simulink library "csu_exr_execute_rts_lib"  (R2014b)
settings: Solver=ode45  StartTime=0.0  StopTime=10.0  RelTol=1e-3
values from neighbouring files (symbols this model uses):
  fsw_dt = 0.02    [csc_sc_wsim_stored_command_test.m]
libraries: simulink x4, util_common_lib x2, util_event_lib x2, util_info_lib x1
settings Model: Creator=escrane  LastModifiedBy=mstewart

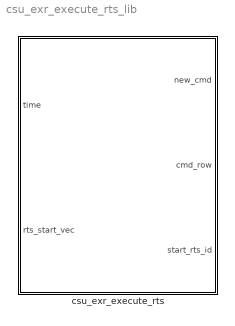
== system csu_exr_execute_rts_lib ==
  csu_exr_execute_rts : Subsystem  mask{rts_id=0, rts_tbl_cmd_time=0, rts_tbl_cmd_data=0}
      mask prompts: rts_id "RTS ID NUMBER"; rts_tbl_cmd_time "RTS CMD TIME"; rts_tbl_cmd_data "RTS CMD DATA"
      mask Display: disp(['RTS #' num2str(rts_id)]);

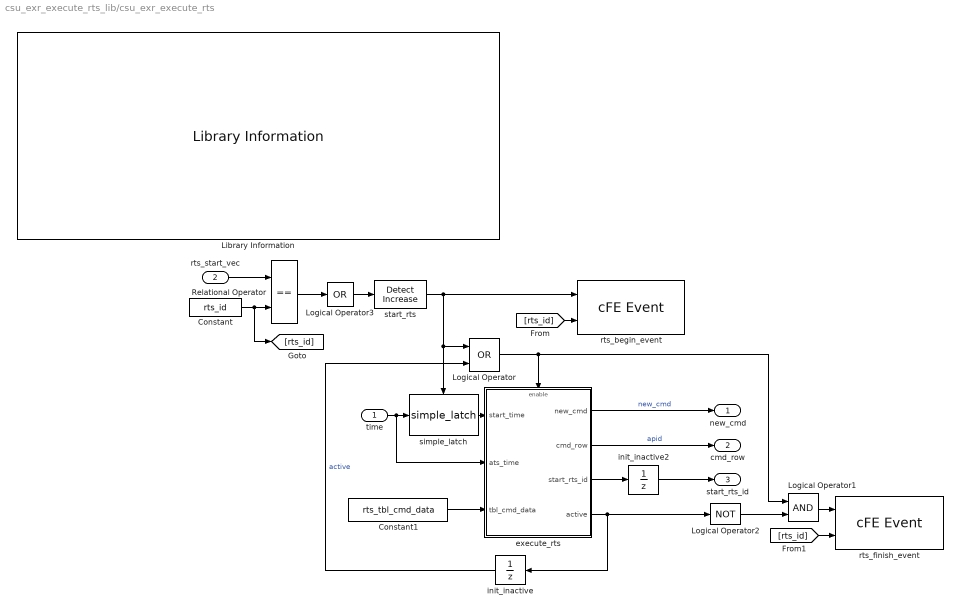
== system csu_exr_execute_rts_lib/csu_exr_execute_rts ==
  time : Inport
  rts_start_vec : Inport  Port=2
  Constant : Constant  Value=rts_id  OutDataTypeStr=uint8
  Constant1 : Constant  Value=rts_tbl_cmd_data  OutDataTypeStr=uint8
  Library Information : util_info_lib/Library Information  owner='escrane'
  Logical Operator : Logic  Operator=OR  AllPortsSameDT=off  OutDataTypeStr=boolean
  Logical Operator1 : Logic  AllPortsSameDT=off  OutDataTypeStr=boolean
  Logical Operator2 : Logic  Operator=NOT  Inputs=1  AllPortsSameDT=off  OutDataTypeStr=boolean
  Logical Operator3 : Logic  Operator=OR  Inputs=1  AllPortsSameDT=off  OutDataTypeStr=boolean
  Relational Operator : RelationalOperator  Operator===  OutDataTypeStr=boolean
  execute_rts : Subsystem  TreatAsAtomicUnit=on
  init_inactive : UnitDelay  SampleTime=-1
  init_inactive2 : UnitDelay  SampleTime=-1
  rts_begin_event : util_event_lib/cFE Event  event_message='Starting RTS #%u'  event_id=20  event_severity=INFORMATION  event_use_enums=off  event_enum_types={}
  rts_finish_event : util_event_lib/cFE Event  event_message='Completed RTS #%u'  event_id=21  event_severity=INFORMATION  event_use_enums=off  event_enum_types={}
  simple_latch : util_common_lib/simple_latch  SystemSampleTime=-1
  start_rts : simulink/Logic and Bit Operations/Detect Increase  vinit=0.0  InputProcessing=Inherited  OutDataTypeStr=boolean
  new_cmd : Outport
  cmd_row : Outport  Port=2
  start_rts_id : Outport  Port=3
  wires:
  init_inactive2/1 -> start_rts_id/1
  execute_rts/3(start_rts_id) -> init_inactive2/1
  Logical Operator3/1 -> start_rts/1
  init_inactive/1 -> Logical Operator/2  "active"
  Constant1/1 -> execute_rts/3(tbl_cmd_data)
  start_rts/1 -> rts_begin_event/1, simple_latch/Trigger, Logical Operator/1
  Logical Operator/1 -> Logical Operator1/1, execute_rts/Enable
  execute_rts/1(new_cmd) -> new_cmd/1  "new_cmd"
  Relational Operator/1 -> Logical Operator3/1
  time/1 -> simple_latch/1, execute_rts/2(ats_time)
  simple_latch/1 -> execute_rts/1(start_time)
  execute_rts/2(cmd_row) -> cmd_row/1  "apid"
  rts_start_vec/1 -> Relational Operator/1
  [rts_id] -> rts_begin_event/2
  Constant/1 -> [rts_id], Relational Operator/2
  [rts_id] -> rts_finish_event/2
  Logical Operator1/1 -> rts_finish_event/1
  execute_rts/4(active) -> Logical Operator2/1, init_inactive/1
  Logical Operator2/1 -> Logical Operator1/2

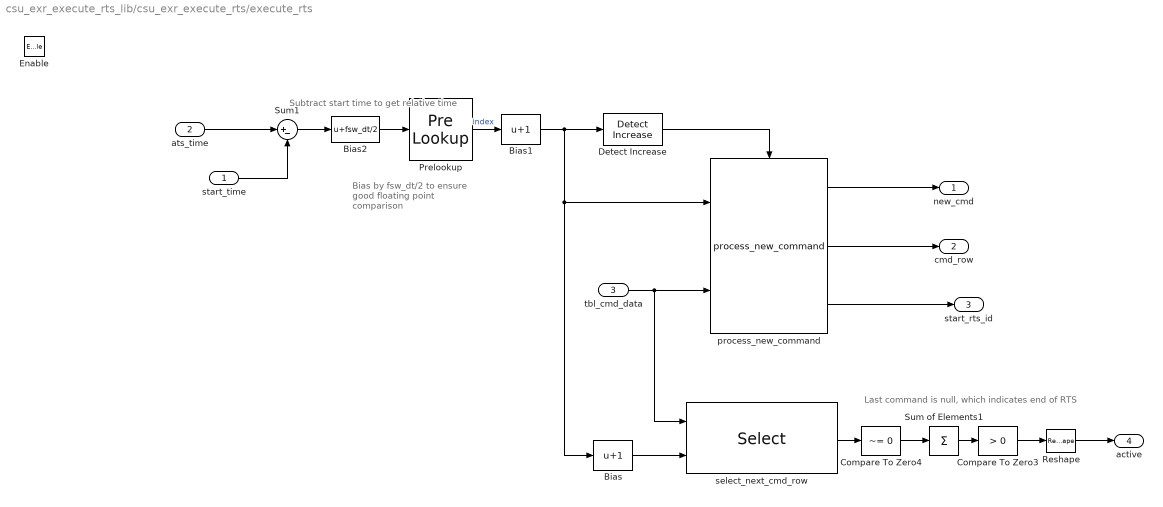
== system csu_exr_execute_rts_lib/csu_exr_execute_rts/execute_rts ==
  note: Bias by fsw_dt/2
      | to ensure good floating
      | point comparison
  note: Last command is null, which indicates end of RTS
  note: Subtract start time to get relative time
  start_time : Inport
  ats_time : Inport  Port=2
  tbl_cmd_data : Inport  Port=3
  Enable : EnablePort  StatesWhenEnabling=reset
  Bias : Bias  Bias=1  SaturateOnIntegerOverflow=on
  Bias1 : Bias  Bias=1  SaturateOnIntegerOverflow=on
  Bias2 : Bias  Bias=fsw_dt/2  SaturateOnIntegerOverflow=on
  Compare To Zero3 : simulink/Logic and Bit Operations/Compare To Zero  relop=>  OutDataTypeStr=uint8
  Compare To Zero4 : simulink/Logic and Bit Operations/Compare To Zero  relop=~=  OutDataTypeStr=uint8
  Detect Increase : simulink/Logic and Bit Operations/Detect Increase  vinit=1  InputProcessing=Inherited  OutDataTypeStr=boolean
  Prelookup : PreLookup  BreakpointsData=rts_tbl_cmd_time  BeginIndexSearchUsingPreviousIndexResult=on  OutputOnlyTheIndex=on  UseLastBreakpoint=on
  Reshape : Reshape
  Sum of Elements1 : Sum  Inputs=+
  Sum1 : Sum  Inputs=|+-
  process_new_command : util_common_lib/process_new_command  SystemSampleTime=-1
  select_next_cmd_row : Selector  NumberOfDimensions=2  InputPortWidth=3  IndexOptions=Index vector (port),Select all  Indices=[1 3],1  OutputSizes=1,1
  new_cmd : Outport  OutputWhenDisabled=reset  InitialOutput=0
  cmd_row : Outport  Port=2
  start_rts_id : Outport  Port=3  OutputWhenDisabled=reset  InitialOutput=0
  active : Outport  Port=4  OutputWhenDisabled=reset  InitialOutput=0
  wires:
  Bias1/1 -> Detect Increase/1, process_new_command/1, Bias/1
  Prelookup/1 -> Bias1/1  "index"
  Sum1/1 -> Bias2/1
  ats_time/1 -> Sum1/1
  Detect Increase/1 -> process_new_command/Enable
  tbl_cmd_data/1 -> process_new_command/2, select_next_cmd_row/1
  Compare To Zero3/1 -> Reshape/1
  Bias/1 -> select_next_cmd_row/2
  select_next_cmd_row/1 -> Compare To Zero4/1
  Compare To Zero4/1 -> Sum of Elements1/1
  Sum of Elements1/1 -> Compare To Zero3/1
  Reshape/1 -> active/1
  process_new_command/1 -> new_cmd/1
  process_new_command/2 -> cmd_row/1
  start_time/1 -> Sum1/2
  process_new_command/3 -> start_rts_id/1
  Bias2/1 -> Prelookup/1
